simulink model "bot_movment"  (R2021a)
settings: Solver=VariableStepAuto  StartTime=0.0  StopTime=10.0  RelTol=1e-3
libraries: arduinomotorcarrierlib x2
settings Model: Creator=mynam  LastModifiedBy=mynam

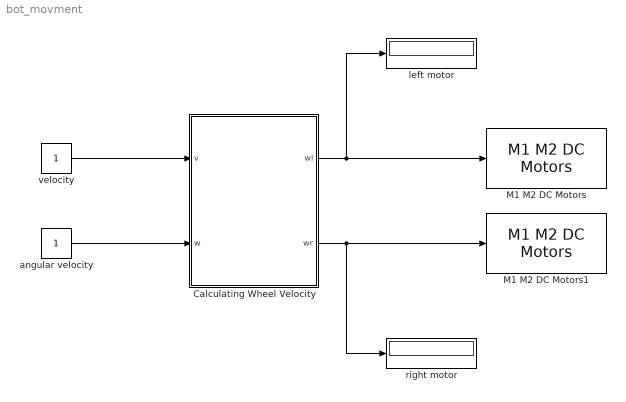
== system bot_movment ==
  Calculating Wheel Velocity : MATLAB Function  TreatAsAtomicUnit=on
  M1 M2 DC Motors : arduinomotorcarrierlib/M1 M2 DC Motors  SlaveAddress=uint8( hex2dec( '66' ) )  blockPlatform=ARDUINO  MotorNumber=M1  MotorCarrierPWMFreq=100
      settings: SourceProductBaseCode=ARDUINO
  M1 M2 DC Motors1 : arduinomotorcarrierlib/M1 M2 DC Motors  SlaveAddress=uint8( hex2dec( '66' ) )  blockPlatform=ARDUINO  MotorNumber=M1  MotorCarrierPWMFreq=100
      settings: SourceProductBaseCode=ARDUINO
  angular velocity : Constant
  left motor : Display
  right motor : Display
  velocity : Constant
  wires:
  velocity/1 -> Calculating Wheel Velocity/1(v)
  angular velocity/1 -> Calculating Wheel Velocity/2(w)
  Calculating Wheel Velocity/1(wl) -> left motor/1, M1 M2 DC Motors/1
  Calculating Wheel Velocity/2(wr) -> M1 M2 DC Motors1/1, right motor/1

== matlab function bot_movment/Calculating Wheel Velocity ==
  data: v input; wl output; w input; wr output
function [wl,wr] = fcn(v,w)
l=8;
r=4;
w=w*pi/180;

wheelVels = 1/r*[1 -l/2; 1 l/2]*[v; w]*180/pi;
wl = wheelVels(1);
wr = wheelVels(2);
